simulink model "myFSK"  (R2019a)
settings: Solver=ode45  StartTime=0.0  StopTime=10.0  RelTol=1e-3  EnableMultiTasking=on
undefined symbols (not defined in the file): fdesignblkfcn, gcbh
libraries: commrandsrc2 x1
settings Model: Creator=Abhishek  LastModifiedBy=JORGE
settings DataIOCC: LimitDataPoints=on  SaveFormat=Array  ReturnWorkspaceOutputs=off
settings OptimizationCC: LifeSpan=inf
settings DebuggingCC: UnderspecifiedInitializationDetection=Classic  MergeDetectMultiDrivingBlocksExec=none  SolverPrmCheckMsg=warning  StateNameClashWarn=warning  SFUnexpectedBacktrackingDiag=warning  SFNoUnconditionalDefaultTransitionDiag=warning  SFExecutionAtInitializationDiag=none  ArithmeticOperatorsInVariantConditions=warning
settings HardwareCC: ProdBitPerPointer=32  ProdBitPerSizeT=32  ProdBitPerPtrDiffT=32  ProdLargestAtomicFloat=None  ProdIntDivRoundTo=Undefined  ProdEndianess=Unspecified  ProdWordSize=32  ProdHWDeviceType=32-bit Generic
settings ModelReferenceCC: PropagateSignalLabelsOutOfModel=off
settings SFSimCC: SimUseLocalCustomCode=off
settings RTWCC: RTWUseLocalCustomCode=off
settings CodeAppCC: StateflowObjectComments=on
settings GRTTargetCC: TargetLangStandard=C89/C90 (ANSI)  GeneratePreprocessorConditionals=Disable all
settings ConfigComp: CovMetricSettings=dw  CovHtmlReporting=on  CovSaveCumulativeToWorkspaceVar=on  CovSaveSingleToWorkspaceVar=on  CovExternalEMLEnable=off

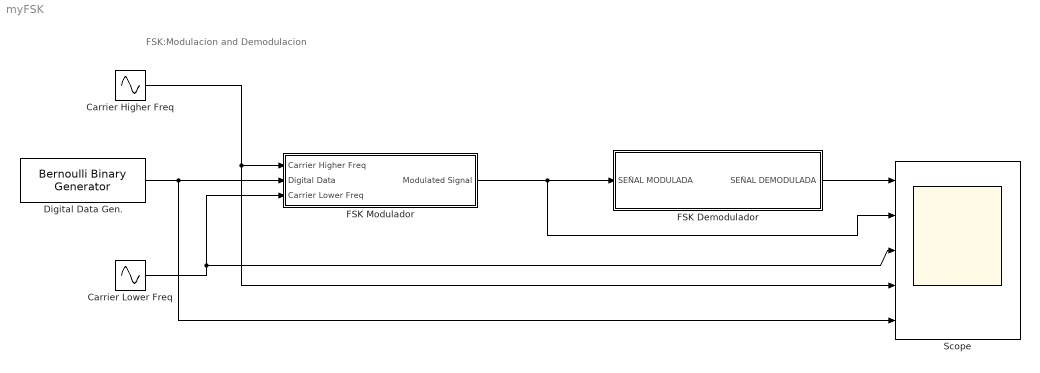
== system myFSK ==
  note: FSK:Modulacion and Demodulacion
  Carrier Higher Freq : Sin  SineType=Sample based  Amplitude=5  Frequency=8*pi  Samples=20  SampleTime=1/100
  Carrier Lower Freq : Sin  SineType=Sample based  Amplitude=5  Frequency=12*pi  Samples=50  SampleTime=1/100
  Digital Data Gen. : commrandsrc2/Bernoulli Binary Generator  P=0.5  seed=61  Ts=1  frameBased=off  sampPerFrame=1  orient=off  outDataType=double  mask(Bernoulli Binary Generator){}
      settings: SourceProductName=Communications Toolbox  SourceProductBaseCode=CM
      mask Display:
      | % This is a new mask on top of the base mask.
      | % Use "View base mask" link below to see the base mask.
      | disp('Digital Msg Signal')
  FSK Demodulador : Subsystem
  FSK Modulador : Subsystem
  "Scope " : Scope  NumInputPorts=5
  wires:
  Digital Data Gen./1 -> "Scope "/5, FSK Modulador/2(Digital Data)
  FSK Modulador/1("Modulated Signal ") -> "Scope "/2, FSK Demodulador/1("SEÑAL MODULADA ")
  Carrier Higher Freq/1 -> "Scope "/4, FSK Modulador/1(Carrier Higher Freq)
  Carrier Lower Freq/1 -> FSK Modulador/3(Carrier Lower Freq), "Scope "/3
  FSK Demodulador/1(SEÑAL DEMODULADA) -> "Scope "/1

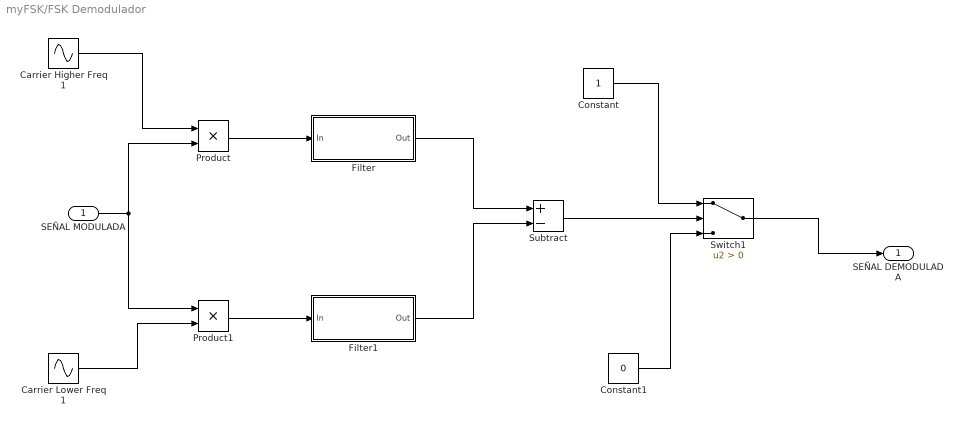
== system myFSK/FSK Demodulador ==
  "SEÑAL MODULADA " : Inport
  Carrier Higher Freq 1 : Sin  SineType=Sample based  Amplitude=5  Frequency=8*pi  Samples=20  SampleTime=1/100
  Carrier Lower Freq 1 : Sin  SineType=Sample based  Amplitude=5  Frequency=12*pi  Samples=50  SampleTime=0.01
  "Constant " : Constant
  "Constant1 " : Constant  Value=0
  Filter : Subsystem  DialogController=fdesignblkfcn  InitFcn=fdesignblkfcn(gcbh, {'InitFcn'});  mask(Lowpass Filter){}
      mask help: Design a lowpass filter
      settings: CopyFcn=fdesignblkfcn(gcbh, {'CopyFcn'});
      mask Help: helpview(mapfilelocation('dsp'), 'dsplowpassfilter');
      mask Display: disp('Lowpass')
  Filter1 : Subsystem  DialogController=fdesignblkfcn  InitFcn=fdesignblkfcn(gcbh, {'InitFcn'});  mask(Lowpass Filter){}
      mask help: Design a lowpass filter
      settings: CopyFcn=fdesignblkfcn(gcbh, {'CopyFcn'});
      mask Help: helpview(mapfilelocation('dsp'), 'dsplowpassfilter');
      mask Display: disp('Lowpass')
  "Product " : Product
  "Product1 " : Product
  "Subtract " : Sum  Inputs=+-
  "Switch1 " : Switch  Criteria=u2 > Threshold
  SEÑAL DEMODULADA : Outport
  wires:
  "SEÑAL MODULADA "/1 -> "Product1 "/1, "Product "/2
  Carrier Higher Freq 1/1 -> "Product "/1
  Carrier Lower Freq 1/1 -> "Product1 "/2
  "Product "/1 -> Filter/1(In)
  "Product1 "/1 -> Filter1/1(In)
  Filter/1(Out) -> "Subtract "/1
  Filter1/1(Out) -> "Subtract "/2
  "Subtract "/1 -> "Switch1 "/2
  "Constant "/1 -> "Switch1 "/1
  "Constant1 "/1 -> "Switch1 "/3
  "Switch1 "/1 -> SEÑAL DEMODULADA/1

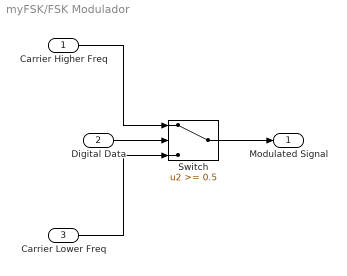
== system myFSK/FSK Modulador ==
  Carrier Higher Freq : Inport
  Digital Data : Inport  Port=2
  Carrier Lower Freq : Inport  Port=3
  "Switch " : Switch  Threshold=0.5
  "Modulated Signal " : Outport
  wires:
  Digital Data/1 -> "Switch "/2
  Carrier Higher Freq/1 -> "Switch "/1
  Carrier Lower Freq/1 -> "Switch "/3
  "Switch "/1 -> "Modulated Signal "/1

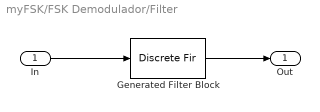
== system myFSK/FSK Demodulador/Filter ==
  In : Inport
  Generated Filter Block : DiscreteFir  Tag=BlockMethodSubSystem  Coefficients=[0.065499579760933527 0.019693301579834822 0.022305613229977754 0.024885344785310987 0.027374519236525979 0.029727760599043418 0.031931726705098085 0.033819966531480228 0.035586674517403494 0.036965196096187043 0.038015348337983333 0.038782404074504173 0.039178627855572606 0.039178627855572606 0.038782404074504173 0.038015348337983333 0.036965196096187043 0.035586674517403494 0.033819966531480228 0.031931726705098085 0.029727760599043418 0.027374519236525979 0.024885344785310987 0.022305613229977754 0.019693301579834822 0.065499579760933527]  InputProcessing=Columns as channels (frame based)
  Out : Outport
  wires:
  In/1 -> Generated Filter Block/1
  Generated Filter Block/1 -> Out/1

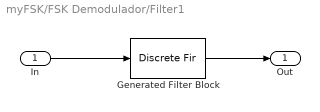
== system myFSK/FSK Demodulador/Filter1 ==
  In : Inport
  Generated Filter Block : DiscreteFir  Tag=BlockMethodSubSystem  Coefficients=[0.065499579760933527 0.019693301579834822 0.022305613229977754 0.024885344785310987 0.027374519236525979 0.029727760599043418 0.031931726705098085 0.033819966531480228 0.035586674517403494 0.036965196096187043 0.038015348337983333 0.038782404074504173 0.039178627855572606 0.039178627855572606 0.038782404074504173 0.038015348337983333 0.036965196096187043 0.035586674517403494 0.033819966531480228 0.031931726705098085 0.029727760599043418 0.027374519236525979 0.024885344785310987 0.022305613229977754 0.019693301579834822 0.065499579760933527]  InputProcessing=Columns as channels (frame based)
  Out : Outport
  wires:
  In/1 -> Generated Filter Block/1
  Generated Filter Block/1 -> Out/1
